simulink model "Modeliranje_i_upravljanje_letjelicom_starter_pack_plain_Usporedbe"  (R2019b)
settings: Solver=VariableStepAuto  StartTime=0.0  StopTime=25.0  RelTol=1e-3
values from neighbouring files (symbols this model uses):
  k_p2 = 1.005572    [Modeliranje_i_upravljanje_letjelicom_starterpack.m]
  k_r2 = 1.001888    [Modeliranje_i_upravljanje_letjelicom_starterpack.m]
  k_y2 = 1.0    (= 1)    [Modeliranje_i_upravljanje_letjelicom_starterpack.m]
  k_z = 6.066    [Modeliranje_i_upravljanje_letjelicom_starterpack.m]
  wn_p2 = 10.672720    (= 10.67272)    [Modeliranje_i_upravljanje_letjelicom_starterpack.m]
  wn_r2 = 12.485386    [Modeliranje_i_upravljanje_letjelicom_starterpack.m]
  wn_y2 = 9.875759    [Modeliranje_i_upravljanje_letjelicom_starterpack.m]
  wn_z = 6.26    [Modeliranje_i_upravljanje_letjelicom_starterpack.m]
  zeta_p2 = 1.000000    (= 1)    [Modeliranje_i_upravljanje_letjelicom_starterpack.m]
  zeta_r2 = 1.000000    (= 1)    [Modeliranje_i_upravljanje_letjelicom_starterpack.m]
  zeta_y2 = 1.000000    (= 1)    [Modeliranje_i_upravljanje_letjelicom_starterpack.m]
settings Model: Creator=Filip  LastModifiedBy=Filip

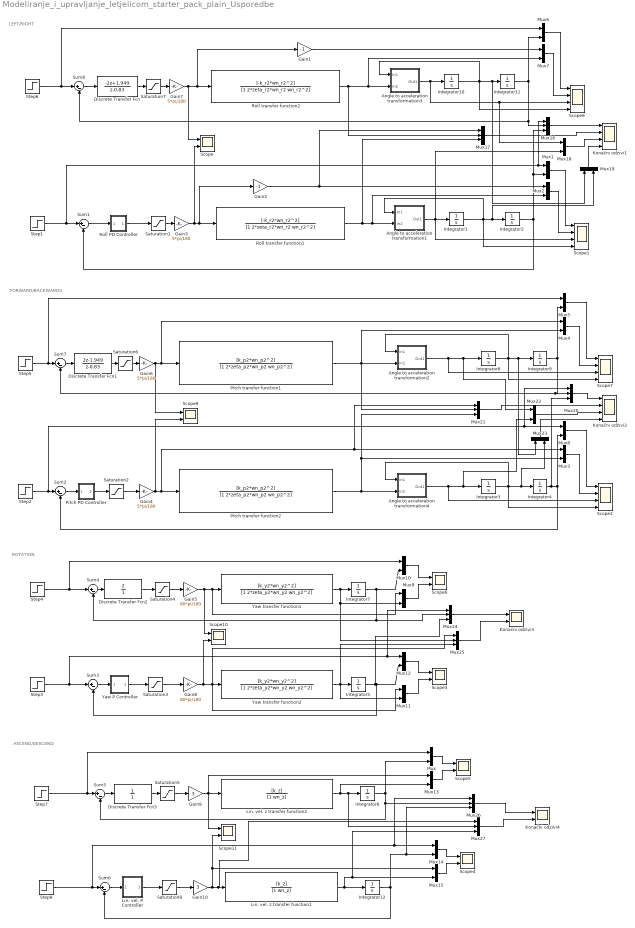
== system Modeliranje_i_upravljanje_letjelicom_starter_pack_plain_Usporedbe ==
  note: LEFT/RIGHT
  note: FORWARD/BACKWARDS
  note: ROTATION
  note: ASCEND/DESCEND
  Angle to acceleration transformation1 : Subsystem
  Angle to acceleration transformation2 : Subsystem
  Angle to acceleration transformation3 : Subsystem
  Angle to acceleration transformation4 : Subsystem
  Discrete Transfer Fcn : DiscreteTransferFcn  Numerator=[-2 1.949]  Denominator=[1 -0.83]  SampleTime=0.04
  Discrete Transfer Fcn1 : DiscreteTransferFcn  Numerator=[2 -1.949]  Denominator=[1 -0.83]  SampleTime=0.04
  Discrete Transfer Fcn2 : DiscreteTransferFcn  Numerator=[2]  Denominator=[1]  SampleTime=0.04
  Discrete Transfer Fcn3 : DiscreteTransferFcn  Denominator=[1]  SampleTime=0.04
  Gain1 : Gain  Gain=-1
  Gain10 : Gain  Gain=3
  Gain2 : Gain  Gain=-1
  Gain{3..4,6..7} (4 alike) : Gain  Gain=5*pi/180
  Gain5 : Gain  Gain=80*pi/180
  Gain8 : Gain  Gain=80*pi/180
  Gain9 : Gain  Gain=3
  Integrator{1..12} (12 alike) : Integrator
  Konačni odzivi1 : Scope  NumInputPorts=4
  Konačni odzivi2 : Scope  NumInputPorts=4
  Konačni odzivi3 : Scope  NumInputPorts=2
  Konačni odzivi4 : Scope  NumInputPorts=2
  Lin. vel. P Controller : Subsystem
  Lin. vel. z transfer function1 : TransferFcn  Numerator=[k_z]  Denominator=[1 wn_z]
  Lin. vel. z transfer function2 : TransferFcn  Numerator=[k_z]  Denominator=[1 wn_z]
  Mux{,1..15,18..19,22..23} (20 alike) : Mux  Inputs=2
  Mux{16..17,20..21,24..27} (8 alike) : Mux  Inputs=3
  Pitch PD Controller : Subsystem
  Pitch transfer function1 : TransferFcn  Numerator=[k_p2*wn_p2^2]  Denominator=[1 2*zeta_p2*wn_p2 wn_p2^2]
  Pitch transfer function2 : TransferFcn  Numerator=[k_p2*wn_p2^2]  Denominator=[1 2*zeta_p2*wn_p2 wn_p2^2]
  Roll PD Controller : Subsystem
  Roll transfer function1 : TransferFcn  Numerator=[-k_r2*wn_r2^2]  Denominator=[1 2*zeta_r2*wn_r2 wn_r2^2]
  Roll transfer function2 : TransferFcn  Numerator=[-k_r2*wn_r2^2]  Denominator=[1 2*zeta_r2*wn_r2 wn_r2^2]
  Saturation{1..8} (8 alike) : Saturate  UpperLimit=1  LowerLimit=-1
  Scope{,3..6,9..11} (8 alike) : Scope  NumInputPorts=2
  Scope{1..2,7..8} (4 alike) : Scope  NumInputPorts=4
  Step1 : Step  Time=0  After=2  SampleTime=0
  Step2 : Step  Time=0  After=2  SampleTime=0
  Step3 : Step  Time=0  After=pi/4  SampleTime=0
  Step4 : Step  Time=0  After=pi/4  SampleTime=0.1
  Step5 : Step  Time=0  After=2  SampleTime=0.1
  Step6 : Step  Time=0  After=2  SampleTime=0.1
  Step7 : Step  Time=0  SampleTime=0.1
  Step8 : Step  Time=0  SampleTime=0
  Sum{1..8} (8 alike) : Sum  Inputs=|+-
  Yaw P Controller : Subsystem
  Yaw transfer function1 : TransferFcn  Numerator=[k_y2*wn_y2^2]  Denominator=[1 2*zeta_y2*wn_y2 wn_y2^2]
  Yaw transfer function2 : TransferFcn  Numerator=[k_y2*wn_y2^2]  Denominator=[1 2*zeta_y2*wn_y2 wn_y2^2]
  wires:
  Mux6/1 -> Scope8/1
  Gain1/1 -> Mux7/1
  Saturation7/1 -> Gain7/1
  Integrator10/1 -> Angle to acceleration transformation3/1(In1), Scope8/4, Mux19/1, Integrator11/1
  Sum8/1 -> Discrete Transfer Fcn/1
  Gain7/1 -> Scope/1, Gain1/1, Roll transfer function2/1
  Discrete Transfer Fcn/1 -> Saturation7/1
  Angle to acceleration transformation3/1(Out1) -> Mux18/1, Scope8/3, Integrator10/1
  Roll transfer function2/1 -> Mux17/2, Mux7/2, Angle to acceleration transformation3/2(In2)
  Mux7/1 -> Scope8/2
  Integrator1/1 -> Angle to acceleration transformation1/1(In1), Scope1/4, Mux19/2, Integrator2/1
  Gain2/1 -> Mux17/1, Mux2/1
  Sum1/1 -> Roll PD Controller/1("  ")
  Mux1/1 -> Scope1/1
  Roll PD Controller/1(" ") -> Saturation1/1
  Mux2/1 -> Scope1/2
  Gain3/1 -> Scope/2, Gain2/1, Roll transfer function1/1
  Step1/1 -> Mux16/1, Mux1/1, Sum1/1
  Saturation1/1 -> Gain3/1
  Roll transfer function1/1 -> Mux17/3, Mux2/2, Angle to acceleration transformation1/2(In2)
  Integrator2/1 -> Mux16/3, Mux1/2, Sum1/2
  Angle to acceleration transformation1/1(Out1) -> Mux18/2, Scope1/3, Integrator1/1
  Discrete Transfer Fcn1/1 -> Saturation6/1
  Sum7/1 -> Discrete Transfer Fcn1/1
  Mux4/1 -> Scope7/2
  Step5/1 -> Mux5/1, Sum7/1
  Saturation6/1 -> Gain6/1
  Pitch transfer function1/1 -> Mux4/2, Angle to acceleration transformation2/2(In2), Mux21/2
  Integrator8/1 -> Angle to acceleration transformation2/1(In1), Scope7/4, Mux23/1, Integrator9/1
  Angle to acceleration transformation2/1(Out1) -> Scope7/3, Mux22/1, Integrator8/1
  Integrator9/1 -> Mux5/2, Mux20/2, Sum7/2
  Mux5/1 -> Scope7/1
  Saturation2/1 -> Gain4/1
  Angle to acceleration transformation4/1(Out1) -> Scope2/3, Mux22/2, Integrator3/1
  Step2/1 -> Mux20/1, Mux8/1, Sum2/1
  Pitch PD Controller/1(" ") -> Saturation2/1
  Integrator3/1 -> Angle to acceleration transformation4/1(In1), Scope2/4, Mux23/2, Integrator4/1
  Pitch transfer function2/1 -> Mux21/3, Mux3/2, Angle to acceleration transformation4/2(In2)
  Integrator4/1 -> Mux20/3, Mux8/2, Sum2/2
  Mux8/1 -> Scope2/1
  Mux3/1 -> Scope2/2
  Sum2/1 -> Pitch PD Controller/1("  ")
  Sum4/1 -> Discrete Transfer Fcn2/1
  Yaw transfer function1/1 -> Mux25/2, Mux9/2, Integrator7/1
  Discrete Transfer Fcn2/1 -> Saturation4/1
  Integrator7/1 -> Mux24/2, Sum4/2, Mux10/2
  Saturation4/1 -> Gain5/1
  Gain5/1 -> Scope10/1, Mux9/1, Yaw transfer function1/1
  Mux9/1 -> Scope6/2
  Step4/1 -> Mux10/1, Sum4/1
  Mux10/1 -> Scope6/1
  Yaw transfer function2/1 -> Mux25/3, Mux11/2, Integrator5/1
  Step3/1 -> Mux24/1, Mux12/1, Sum3/1
  Yaw P Controller/1("  ") -> Saturation3/1
  Gain8/1 -> Scope10/2, Mux25/1, Mux11/1, Yaw transfer function2/1
  Saturation3/1 -> Gain8/1
  Mux12/1 -> Scope3/1
  Mux11/1 -> Scope3/2
  Sum3/1 -> Yaw P Controller/1(" ")
  Discrete Transfer Fcn3/1 -> Saturation5/1
  Gain9/1 -> Scope11/1, Mux13/1, Lin. vel. z transfer function2/1
  Mux13/1 -> Scope5/2
  Integrator6/1 -> Mux/2, Mux26/2, Sum5/2
  Sum5/1 -> Discrete Transfer Fcn3/1
  Mux/1 -> Scope5/1
  Step7/1 -> Mux/1, Sum5/1
  Lin. vel. z transfer function2/1 -> Mux13/2, Mux27/2, Integrator6/1
  Saturation5/1 -> Gain9/1
  Lin. vel. P Controller/1(" ") -> Saturation8/1
  Lin. vel. z transfer function1/1 -> Mux27/3, Mux15/2, Integrator12/1
  Sum6/1 -> Lin. vel. P Controller/1("  ")
  Saturation8/1 -> Gain10/1
  Step8/1 -> Mux26/1, Mux14/1, Sum6/1
  Mux14/1 -> Scope4/1
  Integrator12/1 -> Mux26/3, Mux14/2, Sum6/2
  Mux15/1 -> Scope4/2
  Mux16/1 -> Konačni odzivi1/1
  Integrator11/1 -> Mux16/2, Sum8/2, Mux6/2
  Step6/1 -> Mux6/1, Sum8/1
  Mux17/1 -> Konačni odzivi1/2
  Mux18/1 -> Konačni odzivi1/3
  Mux19/1 -> Konačni odzivi1/4
  Mux20/1 -> Konačni odzivi2/1
  Gain6/1 -> Scope9/1, Mux4/1, Pitch transfer function1/1
  Gain4/1 -> Scope9/2, Mux21/1, Mux3/1, Pitch transfer function2/1
  Mux21/1 -> Konačni odzivi2/2
  Mux22/1 -> Konačni odzivi2/3
  Mux23/1 -> Konačni odzivi2/4
  Mux24/1 -> Konačni odzivi3/1
  Mux25/1 -> Konačni odzivi3/2
  Integrator5/1 -> Sum3/2, Mux12/2, Mux24/3
  Mux26/1 -> Konačni odzivi4/1
  Mux27/1 -> Konačni odzivi4/2
  Gain10/1 -> Scope11/2, Mux15/1, Mux27/1, Lin. vel. z transfer function1/1

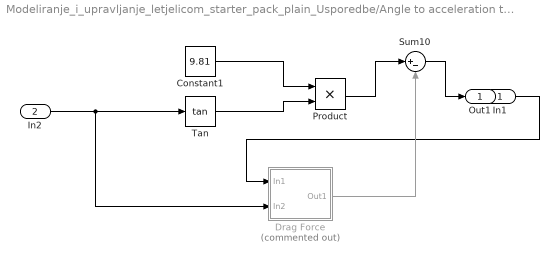
== system Modeliranje_i_upravljanje_letjelicom_starter_pack_plain_Usporedbe/Angle to acceleration transformation1 ==
  In1 : Inport
  In2 : Inport  Port=2
  Constant1 : Constant  Value=9.81
  Drag Force : Subsystem  Commented=on
  Product : Product
  Sum10 : Sum  Inputs=|+-
  Tan : Trigonometry  Operator=tan
  Out1 : Outport
  wires:
  In2/1 -> Drag Force/2(In2), Tan/1
  Constant1/1 -> Product/1
  Tan/1 -> Product/2
  Product/1 -> Sum10/1
  Sum10/1 -> Out1/1
  In1/1 -> Drag Force/1(In1)
  Drag Force/1(Out1) -> Sum10/2

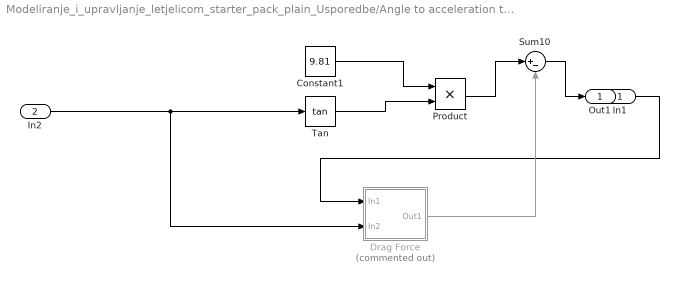
== system Modeliranje_i_upravljanje_letjelicom_starter_pack_plain_Usporedbe/Angle to acceleration transformation2 ==
  In1 : Inport
  In2 : Inport  Port=2
  Constant1 : Constant  Value=9.81
  Drag Force : Subsystem  Commented=on
  Product : Product
  Sum10 : Sum  Inputs=|+-
  Tan : Trigonometry  Operator=tan
  Out1 : Outport
  wires:
  In2/1 -> Drag Force/2(In2), Tan/1
  Sum10/1 -> Out1/1
  Product/1 -> Sum10/1
  Tan/1 -> Product/2
  Constant1/1 -> Product/1
  In1/1 -> Drag Force/1(In1)
  Drag Force/1(Out1) -> Sum10/2

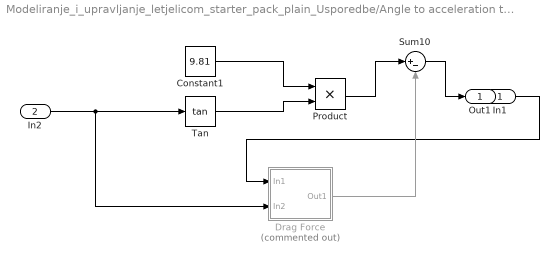
== system Modeliranje_i_upravljanje_letjelicom_starter_pack_plain_Usporedbe/Angle to acceleration transformation3 ==
  In1 : Inport
  In2 : Inport  Port=2
  Constant1 : Constant  Value=9.81
  Drag Force : Subsystem  Commented=on
  Product : Product
  Sum10 : Sum  Inputs=|+-
  Tan : Trigonometry  Operator=tan
  Out1 : Outport
  wires:
  In2/1 -> Drag Force/2(In2), Tan/1
  Constant1/1 -> Product/1
  Tan/1 -> Product/2
  Product/1 -> Sum10/1
  Sum10/1 -> Out1/1
  In1/1 -> Drag Force/1(In1)
  Drag Force/1(Out1) -> Sum10/2

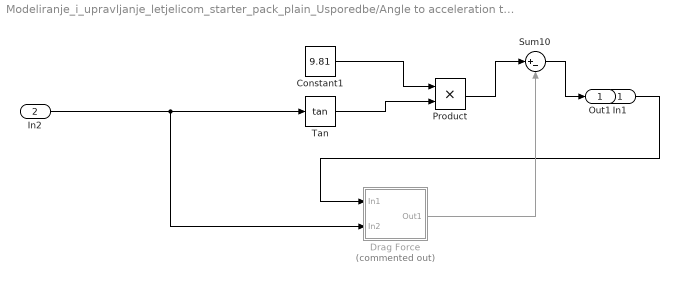
== system Modeliranje_i_upravljanje_letjelicom_starter_pack_plain_Usporedbe/Angle to acceleration transformation4 ==
  In1 : Inport
  In2 : Inport  Port=2
  Constant1 : Constant  Value=9.81
  Drag Force : Subsystem  Commented=on
  Product : Product
  Sum10 : Sum  Inputs=|+-
  Tan : Trigonometry  Operator=tan
  Out1 : Outport
  wires:
  In2/1 -> Drag Force/2(In2), Tan/1
  Sum10/1 -> Out1/1
  Product/1 -> Sum10/1
  Tan/1 -> Product/2
  Constant1/1 -> Product/1
  In1/1 -> Drag Force/1(In1)
  Drag Force/1(Out1) -> Sum10/2

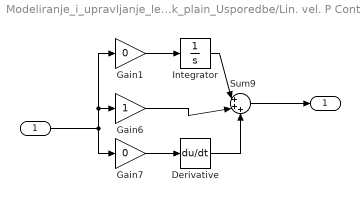
== system Modeliranje_i_upravljanje_letjelicom_starter_pack_plain_Usporedbe/Lin. vel. P Controller ==
  "  " : Inport
  Derivative : Derivative
  Gain1 : Gain  Gain=0
  Gain6 : Gain
  Gain7 : Gain  Gain=0
  Integrator : Integrator
  Sum9 : Sum  Inputs=|+++
  " " : Outport
  wires:
  Sum9/1 -> " "/1
  Gain7/1 -> Derivative/1
  Gain6/1 -> Sum9/2
  Derivative/1 -> Sum9/3
  "  "/1 -> Gain1/1, Gain6/1, Gain7/1
  Integrator/1 -> Sum9/1
  Gain1/1 -> Integrator/1

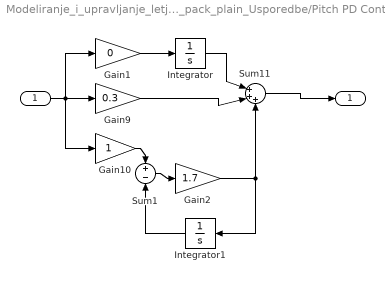
== system Modeliranje_i_upravljanje_letjelicom_starter_pack_plain_Usporedbe/Pitch PD Controller ==
  "  " : Inport
  Gain1 : Gain  Gain=0
  Gain10 : Gain
  Gain2 : Gain  Gain=1.7
  Gain9 : Gain  Gain=0.3
  Integrator : Integrator
  Integrator1 : Integrator
  Sum1 : Sum  Inputs=+-
  Sum11 : Sum  Inputs=|+++
  " " : Outport
  wires:
  Sum11/1 -> " "/1
  "  "/1 -> Gain10/1, Gain1/1, Gain9/1
  Gain10/1 -> Sum1/1
  Gain9/1 -> Sum11/2
  Integrator/1 -> Sum11/1
  Gain1/1 -> Integrator/1
  Sum1/1 -> Gain2/1
  Gain2/1 -> Integrator1/1, Sum11/3
  Integrator1/1 -> Sum1/2

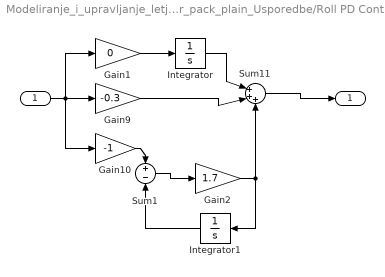
== system Modeliranje_i_upravljanje_letjelicom_starter_pack_plain_Usporedbe/Roll PD Controller ==
  "  " : Inport
  Gain1 : Gain  Gain=0
  Gain10 : Gain  Gain=-1
  Gain2 : Gain  Gain=1.7
  Gain9 : Gain  Gain=-0.3
  Integrator : Integrator
  Integrator1 : Integrator
  Sum1 : Sum  Inputs=+-
  Sum11 : Sum  Inputs=|+++
  " " : Outport
  wires:
  Sum11/1 -> " "/1
  Gain9/1 -> Sum11/2
  "  "/1 -> Gain10/1, Gain1/1, Gain9/1
  Gain1/1 -> Integrator/1
  Gain10/1 -> Sum1/1
  Gain2/1 -> Integrator1/1, Sum11/3
  Integrator/1 -> Sum11/1
  Integrator1/1 -> Sum1/2
  Sum1/1 -> Gain2/1

== system Modeliranje_i_upravljanje_letjelicom_starter_pack_plain_Usporedbe/Yaw P Controller ==
  " " : Inport
  Derivative2 : Derivative
  Gain1 : Gain  Gain=0
  Gain6 : Gain  Gain=0
  Gain7 : Gain  Gain=2
  Integrator : Integrator
  Sum6 : Sum  Inputs=|+++
  "  " : Outport
  wires:
  Sum6/1 -> "  "/1
  Derivative2/1 -> Sum6/3
  " "/1 -> Gain1/1, Gain7/1, Gain6/1
  Gain6/1 -> Derivative2/1
  Gain7/1 -> Sum6/2
  Integrator/1 -> Sum6/1
  Gain1/1 -> Integrator/1

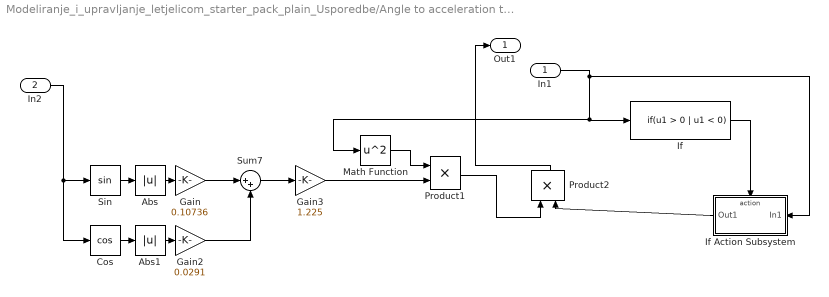
== system Modeliranje_i_upravljanje_letjelicom_starter_pack_plain_Usporedbe/Angle to acceleration transformation1/Drag Force ==
  In1 : Inport
  In2 : Inport  Port=2
  Abs : Abs
  Abs1 : Abs
  Cos : Trigonometry  Operator=cos
  Gain : Gain  Gain=0.10736
  Gain2 : Gain  Gain=0.0291
  Gain3 : Gain  Gain=1.225
  If : If  IfExpression=u1 > 0 | u1 < 0  ShowElse=off
  If Action Subsystem : Subsystem  TreatAsAtomicUnit=on
  Math Function : Math  Operator=square  SignedPower=off  SaturateOnIntegerOverflow=on
  Product1 : Product
  Product2 : Product
  Sin : Trigonometry
  Sum7 : Sum  Inputs=|++
  Out1 : Outport
  wires:
  In1/1 -> If Action Subsystem/1(In1), Math Function/1, If/1
  Cos/1 -> Abs1/1
  Gain3/1 -> Product1/2
  Product2/1 -> Out1/1
  Sum7/1 -> Gain3/1
  In2/1 -> Sin/1, Cos/1
  Abs1/1 -> Gain2/1
  Gain2/1 -> Sum7/2
  Math Function/1 -> Product1/1
  Sin/1 -> Abs/1
  Product1/1 -> Product2/1
  Gain/1 -> Sum7/1
  Abs/1 -> Gain/1
  If/1 -> If Action Subsystem/Action
  If Action Subsystem/1(Out1) -> Product2/2

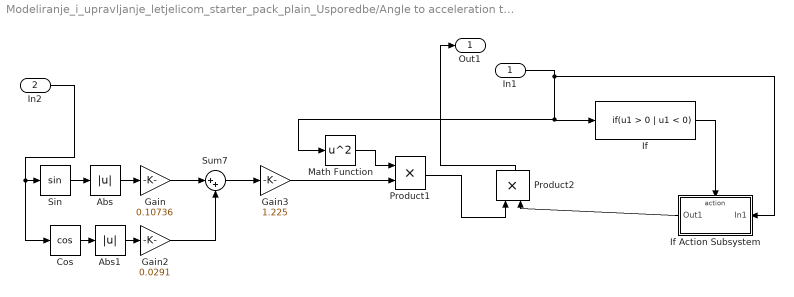
== system Modeliranje_i_upravljanje_letjelicom_starter_pack_plain_Usporedbe/Angle to acceleration transformation2/Drag Force ==
  In1 : Inport
  In2 : Inport  Port=2
  Abs : Abs
  Abs1 : Abs
  Cos : Trigonometry  Operator=cos
  Gain : Gain  Gain=0.10736
  Gain2 : Gain  Gain=0.0291
  Gain3 : Gain  Gain=1.225
  If : If  IfExpression=u1 > 0 | u1 < 0  ShowElse=off
  If Action Subsystem : Subsystem  TreatAsAtomicUnit=on
  Math Function : Math  Operator=square  SignedPower=off  SaturateOnIntegerOverflow=on
  Product1 : Product
  Product2 : Product
  Sin : Trigonometry
  Sum7 : Sum  Inputs=|++
  Out1 : Outport
  wires:
  Cos/1 -> Abs1/1
  Abs/1 -> Gain/1
  Sum7/1 -> Gain3/1
  In1/1 -> If/1, Math Function/1, If Action Subsystem/1(In1)
  If Action Subsystem/1(Out1) -> Product2/2
  Sin/1 -> Abs/1
  In2/1 -> Sin/1, Cos/1
  Gain2/1 -> Sum7/2
  Math Function/1 -> Product1/1
  Abs1/1 -> Gain2/1
  Product1/1 -> Product2/1
  If/1 -> If Action Subsystem/Action
  Gain3/1 -> Product1/2
  Gain/1 -> Sum7/1
  Product2/1 -> Out1/1

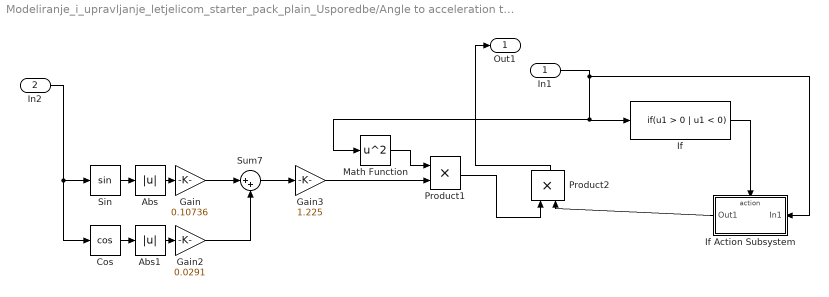
== system Modeliranje_i_upravljanje_letjelicom_starter_pack_plain_Usporedbe/Angle to acceleration transformation3/Drag Force ==
  In1 : Inport
  In2 : Inport  Port=2
  Abs : Abs
  Abs1 : Abs
  Cos : Trigonometry  Operator=cos
  Gain : Gain  Gain=0.10736
  Gain2 : Gain  Gain=0.0291
  Gain3 : Gain  Gain=1.225
  If : If  IfExpression=u1 > 0 | u1 < 0  ShowElse=off
  If Action Subsystem : Subsystem  TreatAsAtomicUnit=on
  Math Function : Math  Operator=square  SignedPower=off  SaturateOnIntegerOverflow=on
  Product1 : Product
  Product2 : Product
  Sin : Trigonometry
  Sum7 : Sum  Inputs=|++
  Out1 : Outport
  wires:
  In1/1 -> If Action Subsystem/1(In1), Math Function/1, If/1
  Cos/1 -> Abs1/1
  Gain3/1 -> Product1/2
  Product2/1 -> Out1/1
  Sum7/1 -> Gain3/1
  In2/1 -> Sin/1, Cos/1
  Abs1/1 -> Gain2/1
  Gain2/1 -> Sum7/2
  Math Function/1 -> Product1/1
  Sin/1 -> Abs/1
  Product1/1 -> Product2/1
  Gain/1 -> Sum7/1
  Abs/1 -> Gain/1
  If/1 -> If Action Subsystem/Action
  If Action Subsystem/1(Out1) -> Product2/2

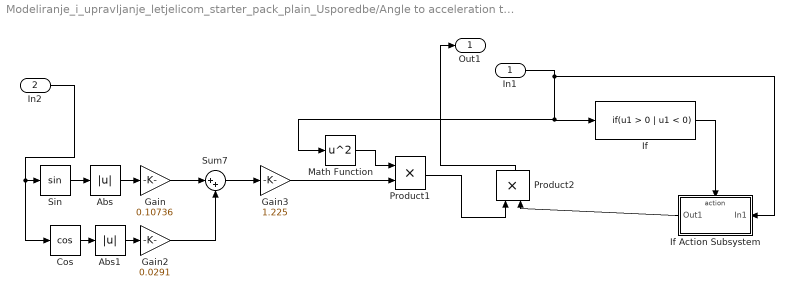
== system Modeliranje_i_upravljanje_letjelicom_starter_pack_plain_Usporedbe/Angle to acceleration transformation4/Drag Force ==
  In1 : Inport
  In2 : Inport  Port=2
  Abs : Abs
  Abs1 : Abs
  Cos : Trigonometry  Operator=cos
  Gain : Gain  Gain=0.10736
  Gain2 : Gain  Gain=0.0291
  Gain3 : Gain  Gain=1.225
  If : If  IfExpression=u1 > 0 | u1 < 0  ShowElse=off
  If Action Subsystem : Subsystem  TreatAsAtomicUnit=on
  Math Function : Math  Operator=square  SignedPower=off  SaturateOnIntegerOverflow=on
  Product1 : Product
  Product2 : Product
  Sin : Trigonometry
  Sum7 : Sum  Inputs=|++
  Out1 : Outport
  wires:
  Cos/1 -> Abs1/1
  Abs/1 -> Gain/1
  Sum7/1 -> Gain3/1
  In1/1 -> If/1, Math Function/1, If Action Subsystem/1(In1)
  If Action Subsystem/1(Out1) -> Product2/2
  Sin/1 -> Abs/1
  In2/1 -> Sin/1, Cos/1
  Gain2/1 -> Sum7/2
  Math Function/1 -> Product1/1
  Abs1/1 -> Gain2/1
  Product1/1 -> Product2/1
  If/1 -> If Action Subsystem/Action
  Gain3/1 -> Product1/2
  Gain/1 -> Sum7/1
  Product2/1 -> Out1/1

== system Modeliranje_i_upravljanje_letjelicom_starter_pack_plain_Usporedbe/Angle to acceleration transformation1/Drag Force/If Action Subsystem ==
  In1 : Inport
  Action Port : ActionPort
  Abs : Abs
  Divide : Product  Inputs=*/
  Out1 : Outport
  wires:
  Abs/1 -> Divide/2
  In1/1 -> Divide/1, Abs/1
  Divide/1 -> Out1/1

== system Modeliranje_i_upravljanje_letjelicom_starter_pack_plain_Usporedbe/Angle to acceleration transformation2/Drag Force/If Action Subsystem ==
  In1 : Inport
  Action Port : ActionPort
  Abs : Abs
  Divide : Product  Inputs=*/
  Out1 : Outport
  wires:
  Divide/1 -> Out1/1
  In1/1 -> Abs/1, Divide/1
  Abs/1 -> Divide/2

== system Modeliranje_i_upravljanje_letjelicom_starter_pack_plain_Usporedbe/Angle to acceleration transformation3/Drag Force/If Action Subsystem ==
  In1 : Inport
  Action Port : ActionPort
  Abs : Abs
  Divide : Product  Inputs=*/
  Out1 : Outport
  wires:
  Abs/1 -> Divide/2
  In1/1 -> Divide/1, Abs/1
  Divide/1 -> Out1/1

== system Modeliranje_i_upravljanje_letjelicom_starter_pack_plain_Usporedbe/Angle to acceleration transformation4/Drag Force/If Action Subsystem ==
  In1 : Inport
  Action Port : ActionPort
  Abs : Abs
  Divide : Product  Inputs=*/
  Out1 : Outport
  wires:
  Divide/1 -> Out1/1
  In1/1 -> Abs/1, Divide/1
  Abs/1 -> Divide/2
